simulink model "antenna_simulation"  (R2015b)
settings: Solver=VariableStepAuto  StartTime=0.0  StopTime=15.0  RelTol=1e-3
libraries: simulink_extras x2
settings Model: Creator=ekin  LastModifiedBy=ekin

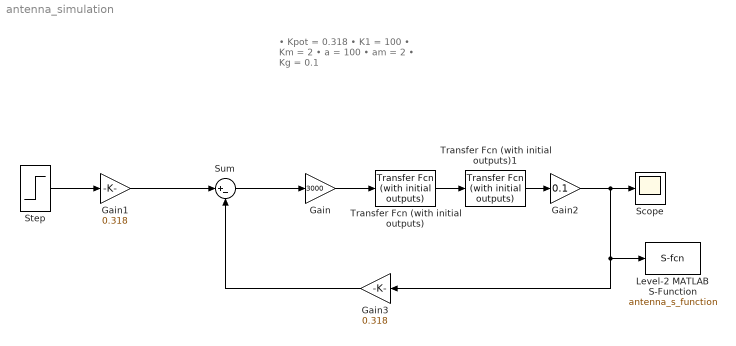
== system antenna_simulation ==
  note: • Kpot = 0.318
      | • K1 = 100
      | • Km = 2
      | • a = 100
      | • am = 2
      | • Kg = 0.1
  Gain : Gain  Gain=3000
  Gain1 : Gain  Gain=0.318
  Gain2 : Gain  Gain=0.1
  Gain3 : Gain  Gain=0.318
  Level-2 MATLAB S-Function : M-S-Function  FunctionName=antenna_s_function
  Scope : Scope
  Step : Step  SampleTime=0
  Sum : Sum  Inputs=|+-
  Transfer Fcn (with initial outputs) : simulink_extras/Additional Linear/Transfer Fcn (with initial outputs)  N=[100]  D="[1  100]"  Y0=0  U0=0
  Transfer Fcn (with initial outputs)1 : simulink_extras/Additional Linear/Transfer Fcn (with initial outputs)  N=[2]  D="[1  2 0]"  Y0=0  U0=0
  wires:
  Gain/1 -> Transfer Fcn (with initial outputs)/1
  Transfer Fcn (with initial outputs)/1 -> Transfer Fcn (with initial outputs)1/1
  Transfer Fcn (with initial outputs)1/1 -> Gain2/1
  Gain2/1 -> Level-2 MATLAB S-Function/1, Gain3/1, Scope/1
  Step/1 -> Gain1/1
  Gain1/1 -> Sum/1
  Gain3/1 -> Sum/2
  Sum/1 -> Gain/1
